simulink model "Malata_Problem7"  (R2023b)
settings: Solver=VariableStepAuto  StartTime=0.0  StopTime=20  RelTol=1e-3
values from neighbouring files (symbols this model uses):
  G_den7 = [1 2 3 4 5 1]    [Malata_Problem7and8.m]    (also in Problem7and8.m)
  G_num7 = [6 5 4 3 2]    [Malata_Problem7and8.m]    (also in Problem7and8.m)
settings Model: Creator=Asus  LastModifiedBy=Rei

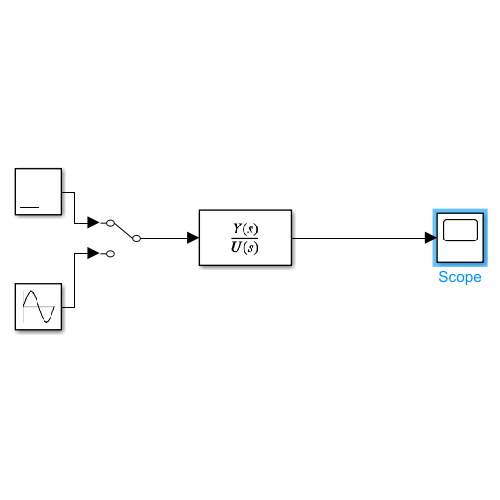
[thumbnail: Simulink's stored preview of the top-level diagram]
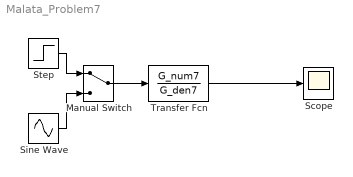
== system Malata_Problem7 ==
  Manual Switch : ManualSwitch
  Scope : Scope
  Sine Wave : Sin  SampleTime=0
  Step : Step  Time=0  SampleTime=0
  Transfer Fcn : TransferFcn  Numerator=G_num7  Denominator=G_den7
  wires:
  Step/1 -> Manual Switch/1
  Sine Wave/1 -> Manual Switch/2
  Manual Switch/1 -> Transfer Fcn/1
  Transfer Fcn/1 -> Scope/1
